simulink model "INtegrated_Simplified_Batteries_2"  (R2025a)
settings: Solver=ode113  StartTime=0.0  StopTime=20000  FixedStep=0.01  MaxStep=0.1  RelTol=1e-3
libraries: simulink x16, slpidlib x2, spsFirstOrderFilterLib x1
(part 1 of 3)
settings Model: Creator=kbiswas  LastModifiedBy=kaust
settings SolverCC: ZeroCrossAlgorithm=Adaptive
settings DebuggingCC: UnderspecifiedInitializationDetection=Classic  MergeDetectMultiDrivingBlocksExec=none
settings ModelReferenceCC: PropagateSignalLabelsOutOfModel=off
settings RTWCC: GPUComputeCapability=3.5

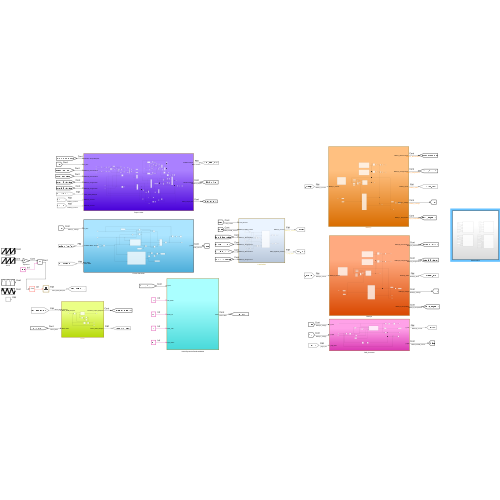
[thumbnail: Simulink's stored preview of the top-level diagram]
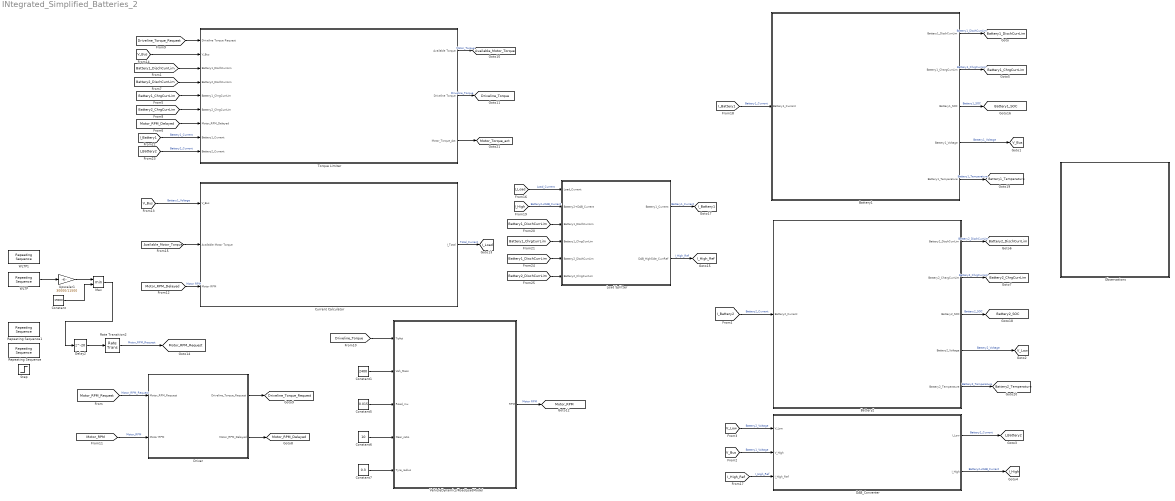
== system INtegrated_Simplified_Batteries_2 ==
  Battery1 : Subsystem
  Battery2 : Subsystem
  Constant : Constant  Value=19000
  Constant1 : Constant  Value=2400
  Constant5 : Constant  Value=0.015
  Constant6 : Constant  Value=10
  Constant7 : Constant  Value=0.3
  Current Calculator : Subsystem
  DAB_Converter : Subsystem
  Delay2 : Delay  DelayLength=20
  Driver : Subsystem
  Load Splitter : Subsystem
  Max : MinMax  Inputs=2
  Observations : Subsystem
  Rate Transition2 : RateTransition
  Repeating Sequence : simulink/Sources/Repeating Sequence  rep_seq_t=[0 20 40 60 80]  rep_seq_y=[0 16000 0 -16000 0]
  Repeating Sequence1 : simulink/Sources/Repeating Sequence  rep_seq_t=[0 0.5 1 2 4 8 16 22 30 38 44 52 56 58 59 59.5 60 64]  rep_seq_y=[0 200 1000 4000 10000 12000 15500 17000 17500 17000 15500 12000 10000 4000 1000 500 0 0]
  Step : Step  Time=2  After=6000  SampleTime=0
  Torque Limiter : Subsystem
  Upscaler1 : Gain  Gain=30000/11500
  VehicleDynamics/RoadLoadModel : Subsystem
  WLTP : simulink/Sources/Repeating Sequence  rep_seq_t=time  rep_seq_y=WLTP_data
  WLTP1 : simulink/Sources/Repeating Sequence  rep_seq_t=time  rep_seq_y=WLTP_data
  tag scope: Available_Motor_Torque=global, Battery1_ChrgCurrLim=global, Battery1_DischCurrLim=global, Battery1_SOC=global, Battery1_Temperature=global, Battery2_ChrgCurrLim=global, Battery2_DischCurrLim=global, Battery2_SOC=global, Battery2_Temperature=global, Driveline_Torque=global, Driveline_Torque_Request=global, I_Battery1=global, I_Battery2=global, I_High=global, I_High_Ref=global, I_Load=global, Motor_RPM=global, Motor_RPM_Delayed=global, Motor_RPM_Request=global, Motor_Torque_act=global, V_Bus=global, V_Low=global
  wires:
  Battery1/1(Battery1_DischCurrLim) -> [Battery1_DischCurrLim]  "Battery1_DischCurrLim"
  Battery1/2(Battery1_ChargCurrLim) -> [Battery1_ChrgCurrLim]  "Battery1_ChrgCurrLim"
  Battery1/4(Battery1_Voltage) -> [V_Bus]  "Battery1_Voltage"
  Battery2/1(Battery2_DischCurrLim) -> [Battery2_DischCurrLim]  "Battery2_DischCurrLim"
  Battery2/2(Battery2_ChargCurrLim) -> [Battery2_ChrgCurrLim]  "Battery2_ChrgCurrLim"
  Battery2/4(Battery2_Voltage) -> [V_Low]  "Battery2_Voltage"
  [I_Battery2] -> Battery2/1(Battery2_Current)  "Battery2_Current"
  [V_Bus] -> DAB_Converter/2(V_High)  "Battery1_Voltage"
  DAB_Converter/1(I_Low) -> [I_Battery2]  "Battery2_Current"
  [V_Low] -> DAB_Converter/1(V_Low)  "Battery2_Voltage"
  [I_Load] -> Load Splitter/1(Load_Current)  "Load_Current"
  DAB_Converter/2(I_High) -> [I_High]  "Battery2+DAB_Current"
  [Motor_RPM_Delayed] -> Current Calculator/3(Motor RPM)  "Motor RPM"
  Torque Limiter/2(Driveline Torque) -> [Driveline_Torque]  "Driveline_Torque"
  [Motor_RPM] -> Driver/2(Motor RPM)  "Motor_RPM"
  [Motor_RPM_Request] -> Driver/1(Motor_RPM_Request)  "Motor_RPM_Request"
  Driver/1(Driveline_Torque_Request) -> [Driveline_Torque_Request]
  [Available_Motor_Torque] -> Current Calculator/2(Available Motor Torque)
  [Battery2_ChrgCurrLim] -> Torque Limiter/6(Battery2_ChrgCurrLim)
  [Driveline_Torque] -> VehicleDynamics/RoadLoadModel/1(TqAct)
  [V_Bus] -> Torque Limiter/2(V_Bus)
  [Battery1_ChrgCurrLim] -> Torque Limiter/5(Battery1_ChrgCurrLim)
  [Battery1_DischCurrLim] -> Torque Limiter/3(Battery1_DischCurrLim)
  [V_Bus] -> Current Calculator/1(V_Bus)  "Battery1_Voltage"
  Constant6/1 -> VehicleDynamics/RoadLoadModel/4(Gear_ratio)
  Constant1/1 -> VehicleDynamics/RoadLoadModel/2(Veh_Mass)
  Constant5/1 -> VehicleDynamics/RoadLoadModel/3(Road_mu)
  [Battery2_DischCurrLim] -> Torque Limiter/4(Battery2_DischCurrLim)
  [Motor_RPM_Delayed] -> Torque Limiter/7(Motor_RPM_Delayed)
  Torque Limiter/1(Available Torque) -> [Available_Motor_Torque]  "Motor_Torque"
  Constant7/1 -> VehicleDynamics/RoadLoadModel/5(Tyre_radius)
  VehicleDynamics/RoadLoadModel/1(RPM) -> [Motor_RPM]  "Motor RPM"
  Driver/2(Motor_RPM_Delayed) -> [Motor_RPM_Delayed]
  Current Calculator/1(I_Total) -> [I_Load]  "Total_Current"
  [Driveline_Torque_Request] -> Torque Limiter/1(Driveline Torque Request)
  Rate Transition2/1 -> [Motor_RPM_Request]  "Motor_RPM_Request"
  Delay2/1 -> Rate Transition2/1
  [I_High_Ref] -> DAB_Converter/3(I_High_Ref)  "I_High_Ref"
  [I_Battery1] -> Battery1/1(Battery1_Current)  "Battery1_Current"
  Load Splitter/1(Battery1_Current) -> [I_Battery1]  "Battery1_Current"
  Load Splitter/2(DAB_HighSide_CurrRef) -> [I_High_Ref]  "I_High_Ref"
  [I_High] -> Load Splitter/2(Battery2+DAB_Current)  "Battery2+DAB_Current"
  [Battery1_DischCurrLim] -> Load Splitter/3(Battery1_DischCurrLim)
  [Battery1_ChrgCurrLim] -> Load Splitter/4(Battery1_ChrgCurrLim)
  Battery1/3(Battery1_SOC) -> [Battery1_SOC]  "Battery1_SOC"
  Battery2/3(Battery2_SOC) -> [Battery2_SOC]  "Battery2_SOC"
  Battery1/5(Battery1_Temperature) -> [Battery1_Temperature]  "Battery1_Temperature"
  Battery2/5(Battery2_Temperature) -> [Battery2_Temperature]  "Battery2_Temperature"
  [I_Battery1] -> Torque Limiter/8(Battery1_Current)  "Battery1_Current"
  [I_Battery2] -> Torque Limiter/9(Battery2_Current)  "Battery2_Current"
  Torque Limiter/3(Motor_Torque_Act) -> [Motor_Torque_act]
  WLTP/1 -> Upscaler1/1
  Constant/1 -> Max/2
  Max/1 -> Delay2/1
  [Battery2_DischCurrLim] -> Load Splitter/6(Battery2_ChrgCurrLim)
  [Battery1_DischCurrLim] -> Load Splitter/5(Battery2_DischCurrLim)
  Upscaler1/1 -> Max/1

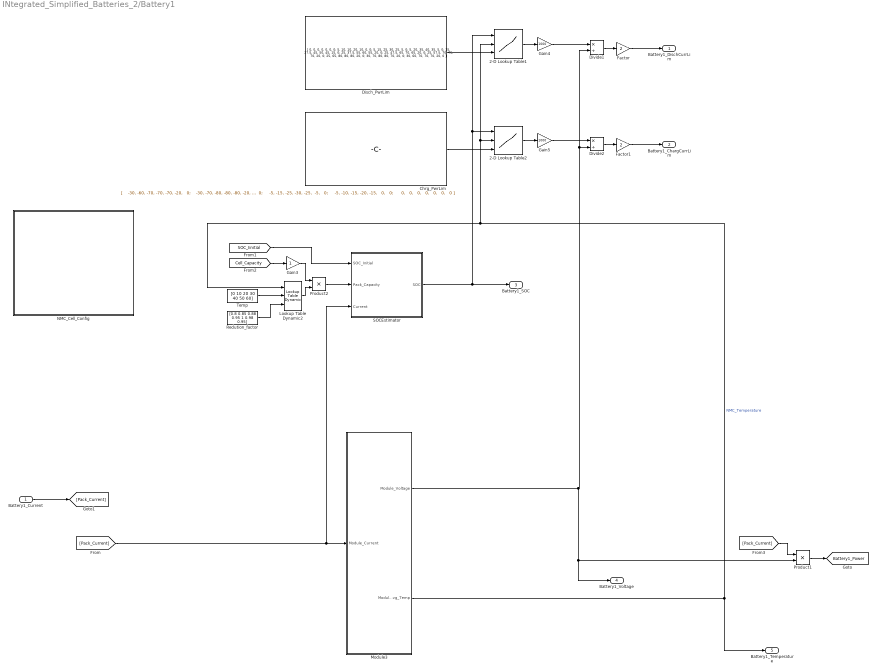
== system INtegrated_Simplified_Batteries_2/Battery1 ==
  Battery1_Current : Inport
  2-D Lookup Table1 : Lookup_n-D  LookupTableObject=''  BreakpointsForDimension1=[0 0.1 0.2 0.3 0.4 0.5 0.6 0.7 0.8 0.9 1]  BreakpointsForDimension2=[0 10 20 30 40 50 60]  BreakpointsForDimension1FirstPoint=10  BreakpointsForDimension2FirstPoint=10  BreakpointsForDimension1Spacing=12  BreakpointsForDimension2Spacing=12  IndexSearchMethod=Evenly spaced points  TableSource=Input port  Table=|  InterpMethod=Akima spline  DiagnosticForOutOfRangeInput=Error  InternalRulePriority=Speed  RndMeth=Simplest
      | [
      |     2.954364, 3.109857, 3.273534, 3.3066, 3.34,    3.3734,  3.20473;
      |     3.122427, 3.286765, 3.459753, 3.4947, 3.53,    3.5653,  3.387035;
      |     3.175499, 3.342631, 3.518559, 3.5541, 3.59,    3.6259,  3.444605;
      |     3.210881, 3.379875, 3.557763, 3.5937, 3.63,    3.6663,  3.482985;
      |     3.237417, 3.407808, 3.587166, 3.6234, 3.66,    3.6966,  3.511777;
      |     3.272799, 3.445052, 3.62637,  3.663,  3.7,     3.737,   3.55015;
      |     3.317026, 3.491066, 3.675375, 3.7125, 3.75,    3.7875,  3.598125;
      |     3.387789, 3.566094, 3.753783, 3.7917, 3.83,    3.8683,  3.674885;
      |     3.467398, 3.649892, 3.841992, 3.8808, 3.92,    3.9592,  3.76124;
      |     3.564697, 3.752313, 3.949803, 3.9897, 4.03,    4.0703,  3.866785;
      |     3.653151, 3.845422, 4.047813, 4.0887, 4.13,    4.1713,  3.962735
      | ]
      settings: InputPortMap=u0,u1,p221
  2-D Lookup Table2 : Lookup_n-D  LookupTableObject=''  BreakpointsForDimension1=[0 0.1 0.2 0.3 0.4 0.5 0.6 0.7 0.8 0.9 1]  BreakpointsForDimension2=[0 10 20 30 40 50 60]  BreakpointsForDimension1FirstPoint=10  BreakpointsForDimension2FirstPoint=10  BreakpointsForDimension1Spacing=12  BreakpointsForDimension2Spacing=12  IndexSearchMethod=Evenly spaced points  TableSource=Input port  Table=|  InterpMethod=Akima spline  DiagnosticForOutOfRangeInput=Error  InternalRulePriority=Speed  RndMeth=Simplest
      | [
      |     2.954364, 3.109857, 3.273534, 3.3066, 3.34,    3.3734,  3.20473;
      |     3.122427, 3.286765, 3.459753, 3.4947, 3.53,    3.5653,  3.387035;
      |     3.175499, 3.342631, 3.518559, 3.5541, 3.59,    3.6259,  3.444605;
      |     3.210881, 3.379875, 3.557763, 3.5937, 3.63,    3.6663,  3.482985;
      |     3.237417, 3.407808, 3.587166, 3.6234, 3.66,    3.6966,  3.511777;
      |     3.272799, 3.445052, 3.62637,  3.663,  3.7,     3.737,   3.55015;
      |     3.317026, 3.491066, 3.675375, 3.7125, 3.75,    3.7875,  3.598125;
      |     3.387789, 3.566094, 3.753783, 3.7917, 3.83,    3.8683,  3.674885;
      |     3.467398, 3.649892, 3.841992, 3.8808, 3.92,    3.9592,  3.76124;
      |     3.564697, 3.752313, 3.949803, 3.9897, 4.03,    4.0703,  3.866785;
      |     3.653151, 3.845422, 4.047813, 4.0887, 4.13,    4.1713,  3.962735
      | ]
      settings: InputPortMap=u0,u1,p221
  Chrg_PwrLim : Constant  Value=|
      | [
      |    -30, -60, -70, -70, -70, -20,   0;
      |    -30, -70, -80, -80, -80, -20,   0;
      |    -25, -65, -80, -80, -80, -20,   0;
      |    -25, -55, -70, -75, -70, -20,   0;
      |    -25, -47.5, -65, -70, -65, -20,  0;
      |    -25, -37.5, -55, -60, -55, -20,  0;
      |    -15, -27.5, -45, -50, -45, -15,  0;
      |     -5, -20, -35, -40, -35,  -5,   0;
      |     -5, -15, -25, -30, -25,  -5,   0;
      |     -5, -10, -15, -20, -15,   0,   0;
      |      0,   0,   0,   0,   0,   0,   0
      | ]
  Disch_PwrLim : Constant  Value=|
      | [
      |      0,   0,   0,   0,   0,   0,   0;
      |      5,  10,  10,  20,  10,   0,   0;
      |      5,  15,  25,  30,  25,   5,   0;
      |      5,  20,  35,  40,  35,   5,   0;
      |     15, 27.5, 45,  50,  45,  15,   0;
      |     25, 37.5, 55,  60,  55,  20,   0;
      |     25, 47.5, 65,  70,  65,  20,   0;
      |     25, 57.5, 70,  75,  70,  20,   0;
      |     25, 65,   80,  80,  80,  20,   0;
      |     30, 70,   80,  80,  70,  20,   0;
      |     30, 60,   70,  70,  70,  20,   0
      | ]
  Divide1 : Product  Inputs=*/
  Divide2 : Product  Inputs=*/
  Factor : Gain  Gain=2
  Factor1 : Gain  Gain=2
  Gain3 : Gain
  Gain4 : Gain  Gain=1000
  Gain5 : Gain  Gain=1000
  Lookup Table Dynamic2 : simulink/Lookup Tables/Lookup Table Dynamic  LookUpMeth=Interpolation-Use End Values  OutDataType=fixdt('double')  OutScaling=[]  OutputDataTypeScalingMode=Specify via dialog  OutDataTypeStr=fixdt('double')  DoSatur=off
  Module3 : Subsystem
  NMC_Cell_Config : Subsystem
  Product1 : Product
  Product2 : Product
  Redution_factor : Constant  Value=[0.8 0.85 0.88 0.95 1 0.98 0.95]
  SOCEstimator : Subsystem  TreatAsAtomicUnit=on
  Temp : Constant  Value=[0 10 20 30 40 50 60]
  Battery1_DischCurrLim : Outport
  Battery1_ChargCurrLim : Outport  Port=2
  Battery1_SOC : Outport  Port=3
  Battery1_Voltage : Outport  Port=4
  Battery1_Temperature : Outport  Port=5
  tag scope: Battery1_Power=global
  wires:
  Product2/1 -> SOCEstimator/2(Pack_Capacity)
  [Pack_Current] -> SOCEstimator/3(Current), Module3/1(Module_Current)
  Divide1/1 -> Factor/1
  Module3/2(Module_avg_Temp) -> Battery1_Temperature/1, 2-D Lookup Table1/2, 2-D Lookup Table2/2, Lookup Table Dynamic2/1  "NMC_Temperature"
  Lookup Table Dynamic2/1 -> Product2/2
  Temp/1 -> Lookup Table Dynamic2/2
  Module3/1(Module_Voltage) -> Divide1/2, Divide2/2, Battery1_Voltage/1, Product1/2
  SOCEstimator/1(SOC) -> Battery1_SOC/1, 2-D Lookup Table2/1, 2-D Lookup Table1/1
  Gain4/1 -> Divide1/1
  2-D Lookup Table1/1 -> Gain4/1
  [SOC_Iinitial] -> SOCEstimator/1(SOC_Initial)
  Divide2/1 -> Factor1/1
  Disch_PwrLim/1 -> 2-D Lookup Table1/3
  2-D Lookup Table2/1 -> Gain5/1
  [Cell_Capacity] -> Gain3/1
  Redution_factor/1 -> Lookup Table Dynamic2/3
  Chrg_PwrLim/1 -> 2-D Lookup Table2/3
  Gain3/1 -> Product2/1
  Gain5/1 -> Divide2/1
  Battery1_Current/1 -> [Pack_Current]
  Factor/1 -> Battery1_DischCurrLim/1
  Factor1/1 -> Battery1_ChargCurrLim/1
  [Pack_Current] -> Product1/1
  Product1/1 -> [Battery1_Power]

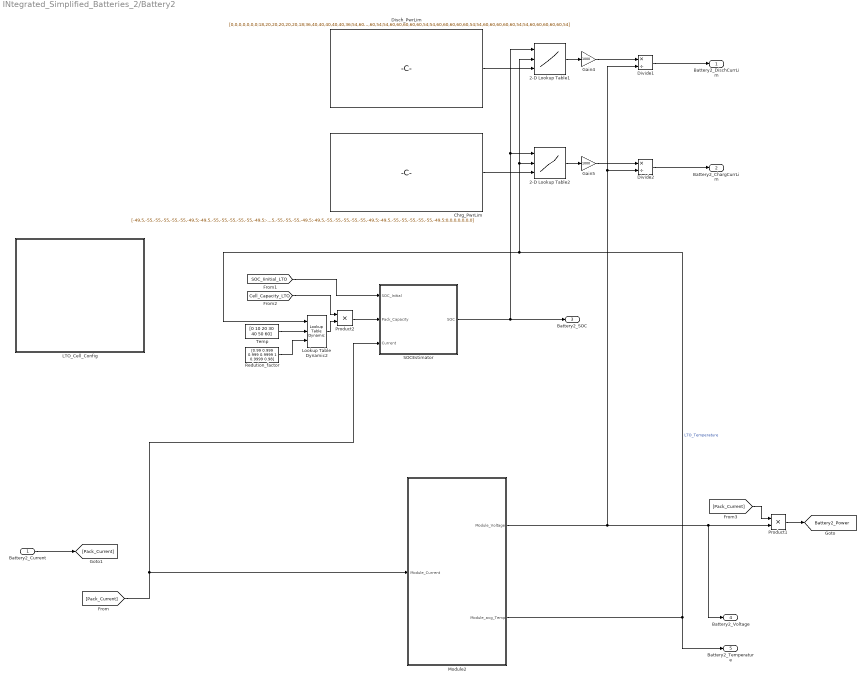
== system INtegrated_Simplified_Batteries_2/Battery2 ==
  Battery2_Current : Inport
  2-D Lookup Table1 : Lookup_n-D  LookupTableObject=''  BreakpointsForDimension1=[0 0.1 0.2 0.3 0.4 0.5 0.6 0.7 0.8 0.9 1]  BreakpointsForDimension2=[0 10 20 30 40 50 60]  BreakpointsForDimension1FirstPoint=10  BreakpointsForDimension2FirstPoint=10  BreakpointsForDimension1Spacing=12  BreakpointsForDimension2Spacing=12  IndexSearchMethod=Evenly spaced points  TableSource=Input port  Table=|  InterpMethod=Akima spline  InternalRulePriority=Speed  RndMeth=Simplest
      | [
      |     2.954364, 3.109857, 3.273534, 3.3066, 3.34,    3.3734,  3.20473;
      |     3.122427, 3.286765, 3.459753, 3.4947, 3.53,    3.5653,  3.387035;
      |     3.175499, 3.342631, 3.518559, 3.5541, 3.59,    3.6259,  3.444605;
      |     3.210881, 3.379875, 3.557763, 3.5937, 3.63,    3.6663,  3.482985;
      |     3.237417, 3.407808, 3.587166, 3.6234, 3.66,    3.6966,  3.511777;
      |     3.272799, 3.445052, 3.62637,  3.663,  3.7,     3.737,   3.55015;
      |     3.317026, 3.491066, 3.675375, 3.7125, 3.75,    3.7875,  3.598125;
      |     3.387789, 3.566094, 3.753783, 3.7917, 3.83,    3.8683,  3.674885;
      |     3.467398, 3.649892, 3.841992, 3.8808, 3.92,    3.9592,  3.76124;
      |     3.564697, 3.752313, 3.949803, 3.9897, 4.03,    4.0703,  3.866785;
      |     3.653151, 3.845422, 4.047813, 4.0887, 4.13,    4.1713,  3.962735
      | ]
      settings: InputPortMap=u0,u1,p221
  2-D Lookup Table2 : Lookup_n-D  LookupTableObject=''  BreakpointsForDimension1=[0 0.1 0.2 0.3 0.4 0.5 0.6 0.7 0.8 0.9 1]  BreakpointsForDimension2=[0 10 20 30 40 50 60]  BreakpointsForDimension1FirstPoint=10  BreakpointsForDimension2FirstPoint=10  BreakpointsForDimension1Spacing=12  BreakpointsForDimension2Spacing=12  IndexSearchMethod=Evenly spaced points  TableSource=Input port  Table=|  InterpMethod=Akima spline  InternalRulePriority=Speed  RndMeth=Simplest
      | [
      |     2.954364, 3.109857, 3.273534, 3.3066, 3.34,    3.3734,  3.20473;
      |     3.122427, 3.286765, 3.459753, 3.4947, 3.53,    3.5653,  3.387035;
      |     3.175499, 3.342631, 3.518559, 3.5541, 3.59,    3.6259,  3.444605;
      |     3.210881, 3.379875, 3.557763, 3.5937, 3.63,    3.6663,  3.482985;
      |     3.237417, 3.407808, 3.587166, 3.6234, 3.66,    3.6966,  3.511777;
      |     3.272799, 3.445052, 3.62637,  3.663,  3.7,     3.737,   3.55015;
      |     3.317026, 3.491066, 3.675375, 3.7125, 3.75,    3.7875,  3.598125;
      |     3.387789, 3.566094, 3.753783, 3.7917, 3.83,    3.8683,  3.674885;
      |     3.467398, 3.649892, 3.841992, 3.8808, 3.92,    3.9592,  3.76124;
      |     3.564697, 3.752313, 3.949803, 3.9897, 4.03,    4.0703,  3.866785;
      |     3.653151, 3.845422, 4.047813, 4.0887, 4.13,    4.1713,  3.962735
      | ]
      settings: InputPortMap=u0,u1,p221
  Chrg_PwrLim : Constant  Value=[-49.5,-55,-55,-55,-55,-55,-49.5;-49.5,-55,-55,-55,-55,-55,-49.5;-49.5,-55,-55,-55,-55,-55,-49.5;-49.5,-55,-55,-55,-55,-55,-49.5;-49.5,-55,-55,-55,-55,-55,-49.5;-49.5,-55,-55,-55,-55,-55,-49.5;-49.5,-55,-55,-55,-55,-55,-49.5;-49.5,-55,-55,-55,-55,-55,-49.5;-49.5,-55,-55,-55,-55,-55,-49.5;-49.5,-55,-55,-55,-55,-55,-49.5;0,0,0,0,0,0,0]
  Disch_PwrLim : Constant  Value=[0,0,0,0,0,0,0;18,20,20,20,20,20,18;36,40,40,40,40,40,36;54,60,60,60,60,60,54;54,60,60,60,60,60,54;54,60,60,60,60,60,54;54,60,60,60,60,60,54;54,60,60,60,60,60,54;54,60,60,60,60,60,54;54,60,60,60,60,60,54;54,60,60,60,60,60,54]
  Divide1 : Product  Inputs=*/
  Divide2 : Product  Inputs=*/
  Gain4 : Gain  Gain=1000
  Gain5 : Gain  Gain=1000
  LTO_Cell_Config : Subsystem
  Lookup Table Dynamic2 : simulink/Lookup Tables/Lookup Table Dynamic  LookUpMeth=Interpolation-Use End Values  OutDataType=fixdt('double')  OutScaling=[]  OutputDataTypeScalingMode=Specify via dialog  OutDataTypeStr=fixdt('double')  DoSatur=off
  Module2 : Subsystem
  Product1 : Product
  Product2 : Product
  Redution_factor : Constant  Value=[0.99 0.999 0.999 0.9999 1 0.9999 0.98]
  SOCEstimator : Subsystem  TreatAsAtomicUnit=on
  Temp : Constant  Value=[0 10 20 30 40 50 60]
  Battery2_DischCurrLim : Outport
  Battery2_ChargCurrLim : Outport  Port=2
  Battery2_SOC : Outport  Port=3
  Battery2_Voltage : Outport  Port=4
  Battery2_Temperature : Outport  Port=5
  tag scope: Battery2_Power=global
  wires:
  Product2/1 -> SOCEstimator/2(Pack_Capacity)
  Divide1/1 -> Battery2_DischCurrLim/1
  Module2/2(Module_avg_Temp) -> Battery2_Temperature/1, 2-D Lookup Table1/2, 2-D Lookup Table2/2, Lookup Table Dynamic2/1  "LTO_Temperature"
  Lookup Table Dynamic2/1 -> Product2/2
  Temp/1 -> Lookup Table Dynamic2/2
  SOCEstimator/1(SOC) -> Battery2_SOC/1, 2-D Lookup Table2/1, 2-D Lookup Table1/1
  Gain4/1 -> Divide1/1
  2-D Lookup Table1/1 -> Gain4/1
  [SOC_Iinitial_LTO] -> SOCEstimator/1(SOC_Initial)
  Divide2/1 -> Battery2_ChargCurrLim/1
  Disch_PwrLim/1 -> 2-D Lookup Table1/3
  2-D Lookup Table2/1 -> Gain5/1
  Redution_factor/1 -> Lookup Table Dynamic2/3
  Chrg_PwrLim/1 -> 2-D Lookup Table2/3
  [Cell_Capacity_LTO] -> Product2/1
  Gain5/1 -> Divide2/1
  Battery2_Current/1 -> [Pack_Current]
  [Pack_Current] -> Module2/1(Module_Current), SOCEstimator/3(Current)
  Module2/1(Module_Voltage) -> Battery2_Voltage/1, Product1/2, Divide2/2, Divide1/2
  [Pack_Current] -> Product1/1
  Product1/1 -> [Battery2_Power]

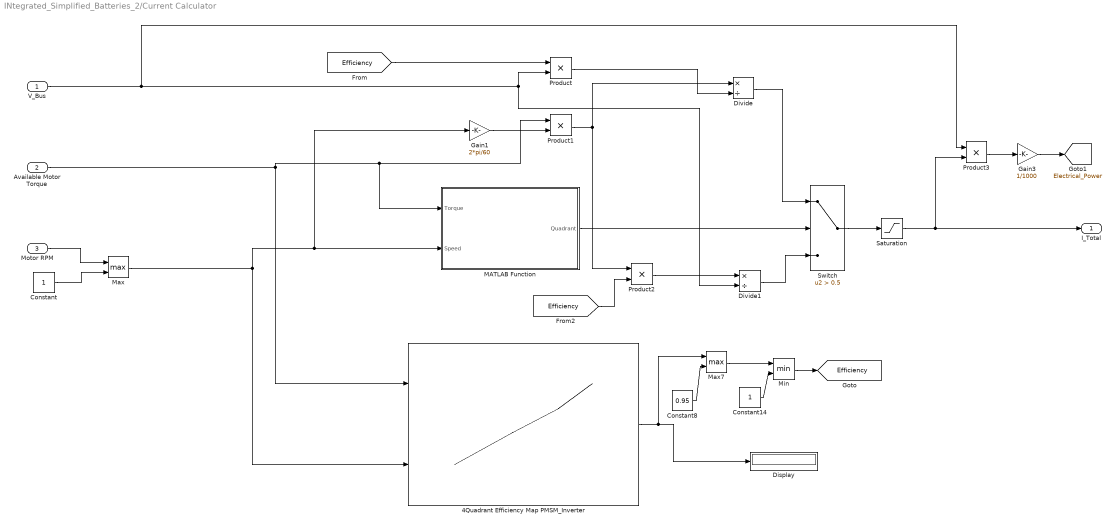
== system INtegrated_Simplified_Batteries_2/Current Calculator ==
  V_Bus : Inport
  Available Motor Torque : Inport  Port=2
  Motor RPM : Inport  Port=3
  4Quadrant Efficiency Map PMSM_Inverter : Lookup_n-D  BreakpointsForDimension1=-200:20:200  BreakpointsForDimension2=-16000:500:16000  Table=|  InterpMethod=Akima spline  InternalRulePriority=Speed  RndMeth=Simplest
      | [0.9785 0.9788 0.9792 0.9795 0.9799 0.9800 0.9800 0.9800 0.9800 0.9800 0.9800 0.9800 0.9800 0.9800 0.9800 0.9800 0.9800 0.9800 0.9800 0.9800 0.9800 0.9800 0.9800 0.9794 0.9781 0.9762 0.9737 0.9699 0.9641 0.9542 0.9347 0.8797 0.0000 0.8632 0.9301 0.9520 0.9628 0.9690 0.9730 0.9757 0.9776 0.9789 0.9799 0.9800 0.9800 0.9800 0.9800 0.9800 0.9800 0.9800 0.9800 0.9800 0.9800 0.9800 0.9800 0.9800 0.9800 0.9800 0.9800 0.9798 0.9794 0.9791 0.9787 0.9784 0.9780;
      | 0.9770 0.9774 0.9778 0.9782 0.9786 0.9790 0.9794 0.9797 0.9800 0.9800 0.9800 0.9800 0.9800 0.9800 0.9800 0.9800 0.9800 0.9800 0.9800 0.9800 0.9800 0.9800 0.9800 0.9800 0.9790 0.9774 0.9752 0.9719 0.9667 0.9578 0.9400 0.8894 0.0000 0.8756 0.9361 0.9559 0.9655 0.9711 0.9746 0.9769 0.9785 0.9797 0.9800 0.9800 0.9800 0.9800 0.9800 0.9800 0.9800 0.9800 0.9800 0.9800 0.9800 0.9800 0.9800 0.9797 0.9793 0.9789 0.9785 0.9781 0.9777 0.9773 0.9769 0.9764 0.9764;
      | 0.9750 0.9755 0.9760 0.9765 0.9769 0.9774 0.9779 0.9783 0.9787 0.9792 0.9796 0.9799 0.9800 0.9800 0.9800 0.9800 0.9800 0.9800 0.9800 0.9800 0.9800 0.9800 0.9800 0.9800 0.9797 0.9785 0.9766 0.9737 0.9691 0.9612 0.9452 0.8992 0.0000 0.8878 0.9420 0.9596 0.9681 0.9730 0.9760 0.9780 0.9793 0.9800 0.9800 0.9800 0.9800 0.9800 0.9800 0.9800 0.9800 0.9800 0.9800 0.9800 0.9799 0.9795 0.9791 0.9787 0.9783 0.9778 0.9774 0.9769 0.9764 0.9759 0.9754 0.9749 0.9743;
      | 0.9723 0.9729 0.9735 0.9741 0.9747 0.9752 0.9758 0.9764 0.9769 0.9774 0.9779 0.9784 0.9789 0.9793 0.9798 0.9800 0.9800 0.9800 0.9800 0.9800 0.9800 0.9800 0.9800 0.9800 0.9800 0.9793 0.9778 0.9754 0.9714 0.9645 0.9503 0.9089 0.0000 0.8998 0.9477 0.9632 0.9706 0.9747 0.9772 0.9788 0.9799 0.9800 0.9800 0.9800 0.9800 0.9800 0.9800 0.9800 0.9800 0.9798 0.9794 0.9789 0.9784 0.9779 0.9774 0.9769 0.9763 0.9758 0.9752 0.9746 0.9740 0.9734 0.9728 0.9722 0.9716;
      | 0.9687 0.9694 0.9701 0.9708 0.9715 0.9722 0.9729 0.9736 0.9743 0.9749 0.9756 0.9762 0.9768 0.9774 0.9780 0.9785 0.9790 0.9795 0.9799 0.9800 0.9800 0.9800 0.9800 0.9800 0.9800 0.9798 0.9786 0.9767 0.9735 0.9676 0.9553 0.9186 0.0000 0.9114 0.9532 0.9665 0.9728 0.9762 0.9782 0.9794 0.9800 0.9800 0.9800 0.9800 0.9800 0.9799 0.9795 0.9791 0.9786 0.9780 0.9775 0.9769 0.9763 0.9756 0.9750 0.9743 0.9736 0.9729 0.9722 0.9714 0.9707 0.9700 0.9692 0.9685 0.9677;
      | 0.9635 0.9644 0.9653 0.9661 0.9670 0.9679 0.9687 0.9696 0.9704 0.9712 0.9721 0.9729 0.9737 0.9744 0.9752 0.9759 0.9767 0.9773 0.9780 0.9786 0.9791 0.9795 0.9798 0.9800 0.9800 0.9798 0.9790 0.9777 0.9751 0.9703 0.9598 0.9280 0.0000 0.9224 0.9582 0.9694 0.9745 0.9772 0.9786 0.9793 0.9796 0.9796 0.9794 0.9791 0.9786 0.9781 0.9775 0.9768 0.9761 0.9753 0.9746 0.9738 0.9730 0.9721 0.9713 0.9704 0.9695 0.9686 0.9677 0.9668 0.9659 0.9649 0.9640 0.9631 0.9621;
      | 0.9557 0.9568 0.9579 0.9590 0.9601 0.9611 0.9622 0.9633 0.9644 0.9655 0.9666 0.9676 0.9687 0.9697 0.9707 0.9717 0.9727 0.9737 0.9746 0.9755 0.9763 0.9771 0.9777 0.9783 0.9787 0.9788 0.9786 0.9778 0.9761 0.9723 0.9638 0.9367 0.0000 0.9324 0.9624 0.9715 0.9755 0.9773 0.9781 0.9784 0.9782 0.9778 0.9772 0.9765 0.9757 0.9749 0.9739 0.9730 0.9720 0.9709 0.9699 0.9688 0.9677 0.9665 0.9654 0.9643 0.9631 0.9619 0.9608 0.9596 0.9584 0.9572 0.9560 0.9548 0.9536;
      | 0.9426 0.9440 0.9455 0.9470 0.9484 0.9499 0.9513 0.9528 0.9543 0.9557 0.9572 0.9586 0.9601 0.9615 0.9629 0.9643 0.9657 0.9671 0.9685 0.9698 0.9710 0.9723 0.9734 0.9745 0.9754 0.9761 0.9765 0.9764 0.9755 0.9730 0.9663 0.9438 0.0000 0.9404 0.9651 0.9722 0.9749 0.9759 0.9759 0.9755 0.9748 0.9738 0.9727 0.9715 0.9702 0.9688 0.9674 0.9660 0.9645 0.9630 0.9615 0.9600 0.9584 0.9568 0.9553 0.9537 0.9521 0.9505 0.9489 0.9472 0.9456 0.9440 0.9424 0.9407 0.9391;
      | 0.9171 0.9192 0.9213 0.9234 0.9256 0.9277 0.9298 0.9320 0.9341 0.9363 0.9384 0.9406 0.9427 0.9449 0.9470 0.9492 0.9513 0.9534 0.9555 0.9576 0.9597 0.9617 0.9637 0.9656 0.9673 0.9689 0.9703 0.9712 0.9714 0.9701 0.9653 0.9463 0.0000 0.9433 0.9640 0.9692 0.9706 0.9703 0.9694 0.9679 0.9662 0.9643 0.9623 0.9602 0.9580 0.9558 0.9535 0.9512 0.9488 0.9464 0.9441 0.9417 0.9392 0.9368 0.9344 0.9319 0.9295 0.9270 0.9245 0.9221 0.9196 0.9171 0.9146 0.9121 0.9096;
      | 0.8478 0.8514 0.8551 0.8588 0.8625 0.8662 0.8700 0.8738 0.8776 0.8815 0.8854 0.8893 0.8932 0.8972 0.9011 0.9051 0.9091 0.9132 0.9172 0.9213 0.9253 0.9293 0.9333 0.9372 0.9410 0.9447 0.9481 0.9510 0.9532 0.9537 0.9502 0.9309 0.0000 0.9257 0.9476 0.9515 0.9509 0.9485 0.9452 0.9415 0.9373 0.9330 0.9285 0.9239 0.9193 0.9145 0.9097 0.9049 0.9001 0.8952 0.8903 0.8854 0.8804 0.8755 0.8705 0.8655 0.8606 0.8556 0.8506 0.8456 0.8406 0.8356 0.8305 0.8255 0.8205;
      | 0.0000 0.0000 0.0000 0.0000 0.0000 0.0000 0.0000 0.0000 0.0000 0.0000 0.0000 0.0000 0.0000 0.0000 0.0000 0.0000 0.0000 0.0000 0.0000 0.0000 0.0000 0.0000 0.0000 0.0000 0.0000 0.0000 0.0000 0.0000 0.0000 0.0000 0.0000 0.0000 0.0000 0.0000 0.0000 0.0000 0.0000 0.0000 0.0000 0.0000 0.0000 0.0000 0.0000 0.0000 0.0000 0.0000 0.0000 0.0000 0.0000 0.0000 0.0000 0.0000 0.0000 0.0000 0.0000 0.0000 0.0000 0.0000 0.0000 0.0000 0.0000 0.0000 0.0000 0.0000 0.0000;
      | 0.8205 0.8255 0.8305 0.8356 0.8406 0.8456 0.8506 0.8556 0.8606 0.8655 0.8705 0.8755 0.8804 0.8854 0.8903 0.8952 0.9001 0.9049 0.9097 0.9145 0.9193 0.9239 0.9285 0.9330 0.9373 0.9415 0.9452 0.9485 0.9509 0.9515 0.9476 0.9257 0.0000 0.9309 0.9502 0.9537 0.9532 0.9510 0.9481 0.9447 0.9410 0.9372 0.9333 0.9293 0.9253 0.9213 0.9172 0.9132 0.9091 0.9051 0.9011 0.8972 0.8932 0.8893 0.8854 0.8815 0.8776 0.8738 0.8700 0.8662 0.8625 0.8588 0.8551 0.8514 0.8478;
      | 0.9096 0.9121 0.9146 0.9171 0.9196 0.9221 0.9245 0.9270 0.9295 0.9319 0.9344 0.9368 0.9392 0.9417 0.9441 0.9464 0.9488 0.9512 0.9535 0.9558 0.9580 0.9602 0.9623 0.9643 0.9662 0.9679 0.9694 0.9703 0.9706 0.9692 0.9640 0.9433 0.0000 0.9463 0.9653 0.9701 0.9714 0.9712 0.9703 0.9689 0.9673 0.9656 0.9637 0.9617 0.9597 0.9576 0.9555 0.9534 0.9513 0.9492 0.9470 0.9449 0.9427 0.9406 0.9384 0.9363 0.9341 0.9320 0.9298 0.9277 0.9256 0.9234 0.9213 0.9192 0.9171;
      | 0.9391 0.9407 0.9424 0.9440 0.9456 0.9472 0.9489 0.9505 0.9521 0.9537 0.9553 0.9568 0.9584 0.9600 0.9615 0.9630 0.9645 0.9660 0.9674 0.9688 0.9702 0.9715 0.9727 0.9738 0.9748 0.9755 0.9759 0.9759 0.9749 0.9722 0.9651 0.9404 0.0000 0.9438 0.9663 0.9730 0.9755 0.9764 0.9765 0.9761 0.9754 0.9745 0.9734 0.9723 0.9710 0.9698 0.9685 0.9671 0.9657 0.9643 0.9629 0.9615 0.9601 0.9586 0.9572 0.9557 0.9543 0.9528 0.9513 0.9499 0.9484 0.9470 0.9455 0.9440 0.9426;
      | 0.9536 0.9548 0.9560 0.9572 0.9584 0.9596 0.9608 0.9619 0.9631 0.9643 0.9654 0.9665 0.9677 0.9688 0.9699 0.9709 0.9720 0.9730 0.9739 0.9749 0.9757 0.9765 0.9772 0.9778 0.9782 0.9784 0.9781 0.9773 0.9755 0.9715 0.9624 0.9324 0.0000 0.9367 0.9638 0.9723 0.9761 0.9778 0.9786 0.9788 0.9787 0.9783 0.9777 0.9771 0.9763 0.9755 0.9746 0.9737 0.9727 0.9717 0.9707 0.9697 0.9687 0.9676 0.9666 0.9655 0.9644 0.9633 0.9622 0.9611 0.9601 0.9590 0.9579 0.9568 0.9557;
      | 0.9621 0.9631 0.9640 0.9649 0.9659 0.9668 0.9677 0.9686 0.9695 0.9704 0.9713 0.9721 0.9730 0.9738 0.9746 0.9753 0.9761 0.9768 0.9775 0.9781 0.9786 0.9791 0.9794 0.9796 0.9796 0.9793 0.9786 0.9772 0.9745 0.9694 0.9582 0.9224 0.0000 0.9280 0.9598 0.9703 0.9751 0.9777 0.9790 0.9798 0.9800 0.9800 0.9798 0.9795 0.9791 0.9786 0.9780 0.9773 0.9767 0.9759 0.9752 0.9744 0.9737 0.9729 0.9721 0.9712 0.9704 0.9696 0.9687 0.9679 0.9670 0.9661 0.9653 0.9644 0.9635;
      | 0.9677 0.9685 0.9692 0.9700 0.9707 0.9714 0.9722 0.9729 0.9736 0.9743 0.9750 0.9756 0.9763 0.9769 0.9775 0.9780 0.9786 0.9791 0.9795 0.9799 0.9800 0.9800 0.9800 0.9800 0.9800 0.9794 0.9782 0.9762 0.9728 0.9665 0.9532 0.9114 0.0000 0.9186 0.9553 0.9676 0.9735 0.9767 0.9786 0.9798 0.9800 0.9800 0.9800 0.9800 0.9800 0.9800 0.9799 0.9795 0.9790 0.9785 0.9780 0.9774 0.9768 0.9762 0.9756 0.9749 0.9743 0.9736 0.9729 0.9722 0.9715 0.9708 0.9701 0.9694 0.9687;
      | 0.9716 0.9722 0.9728 0.9734 0.9740 0.9746 0.9752 0.9758 0.9763 0.9769 0.9774 0.9779 0.9784 0.9789 0.9794 0.9798 0.9800 0.9800 0.9800 0.9800 0.9800 0.9800 0.9800 0.9800 0.9799 0.9788 0.9772 0.9747 0.9706 0.9632 0.9477 0.8998 0.0000 0.9089 0.9503 0.9645 0.9714 0.9754 0.9778 0.9793 0.9800 0.9800 0.9800 0.9800 0.9800 0.9800 0.9800 0.9800 0.9800 0.9800 0.9798 0.9793 0.9789 0.9784 0.9779 0.9774 0.9769 0.9764 0.9758 0.9752 0.9747 0.9741 0.9735 0.9729 0.9723;
      | 0.9743 0.9749 0.9754 0.9759 0.9764 0.9769 0.9774 0.9778 0.9783 0.9787 0.9791 0.9795 0.9799 0.9800 0.9800 0.9800 0.9800 0.9800 0.9800 0.9800 0.9800 0.9800 0.9800 0.9800 0.9793 0.9780 0.9760 0.9730 0.9681 0.9596 0.9420 0.8878 0.0000 0.8992 0.9452 0.9612 0.9691 0.9737 0.9766 0.9785 0.9797 0.9800 0.9800 0.9800 0.9800 0.9800 0.9800 0.9800 0.9800 0.9800 0.9800 0.9800 0.9800 0.9799 0.9796 0.9792 0.9787 0.9783 0.9779 0.9774 0.9769 0.9765 0.9760 0.9755 0.9750;
      | 0.9764 0.9769 0.9773 0.9777 0.9781 0.9785 0.9789 0.9793 0.9797 0.9800 0.9800 0.9800 0.9800 0.9800 0.9800 0.9800 0.9800 0.9800 0.9800 0.9800 0.9800 0.9800 0.9800 0.9797 0.9785 0.9769 0.9746 0.9711 0.9655 0.9559 0.9361 0.8756 0.0000 0.8894 0.9400 0.9578 0.9667 0.9719 0.9752 0.9774 0.9790 0.9800 0.9800 0.9800 0.9800 0.9800 0.9800 0.9800 0.9800 0.9800 0.9800 0.9800 0.9800 0.9800 0.9800 0.9800 0.9800 0.9797 0.9794 0.9790 0.9786 0.9782 0.9778 0.9774 0.9770;
      | 0.9780 0.9784 0.9787 0.9791 0.9794 0.9798 0.9800 0.9800 0.9800 0.9800 0.9800 0.9800 0.9800 0.9800 0.9800 0.9800 0.9800 0.9800 0.9800 0.9800 0.9800 0.9800 0.9799 0.9789 0.9776 0.9757 0.9730 0.9690 0.9628 0.9520 0.9301 0.8632 0.0000 0.8797 0.9347 0.9542 0.9641 0.9699 0.9737 0.9762 0.9781 0.9794 0.9800 0.9800 0.9800 0.9800 0.9800 0.9800 0.9800 0.9800 0.9800 0.9800 0.9800 0.9800 0.9800 0.9800 0.9800 0.9800 0.9800 0.9800 0.9799 0.9795 0.9792 0.9788 0.9785];
      settings: InputPortMap=u0,u1
  Constant : Constant
  Constant14 : Constant
  Constant8 : Constant  Value=0.95
  Display : Display
  Divide : Product  Inputs=*/
  Divide1 : Product  Inputs=*/
  Gain1 : Gain  Gain=2*pi/60
  Gain3 : Gain  Gain=1/1000
  MATLAB Function : MATLAB Function  TreatAsAtomicUnit=on
  Max : MinMax  Function=max  Inputs=2
  Max7 : MinMax  Function=max  Inputs=2
  Min : MinMax  Inputs=2
  Product{,1..3} (4 alike) : Product
  Saturation : Saturate  UpperLimit=400  LowerLimit=-400
  Switch : Switch  Criteria=u2 > Threshold  Threshold=0.5  SaturateOnIntegerOverflow=off  InputSameDT=off
  I_Total : Outport
  tag scope: Efficiency=global, Electrical_Power=global
  wires:
  [Efficiency] -> Product2/2
  Min/1 -> [Efficiency]
  Max/1 -> Gain1/1, MATLAB Function/2(Speed), 4Quadrant Efficiency Map PMSM_Inverter/2
  4Quadrant Efficiency Map PMSM_Inverter/1 -> Max7/1, Display/1
  Max7/1 -> Min/1
  V_Bus/1 -> Product3/1, Product/2, Divide1/2
  Divide/1 -> Switch/1
  Constant14/1 -> Min/2
  [Efficiency] -> Product/1
  Saturation/1 -> Product3/2, I_Total/1
  Available Motor Torque/1 -> Product1/1, MATLAB Function/1(Torque), 4Quadrant Efficiency Map PMSM_Inverter/1
  Constant8/1 -> Max7/2
  Switch/1 -> Saturation/1
  MATLAB Function/1(Quadrant) -> Switch/2
  Product2/1 -> Divide1/1
  Gain1/1 -> Product1/2
  Product1/1 -> Product2/1, Divide/1
  Divide1/1 -> Switch/3
  Product/1 -> Divide/2
  Product3/1 -> Gain3/1
  Gain3/1 -> [Electrical_Power]
  Motor RPM/1 -> Max/1
  Constant/1 -> Max/2

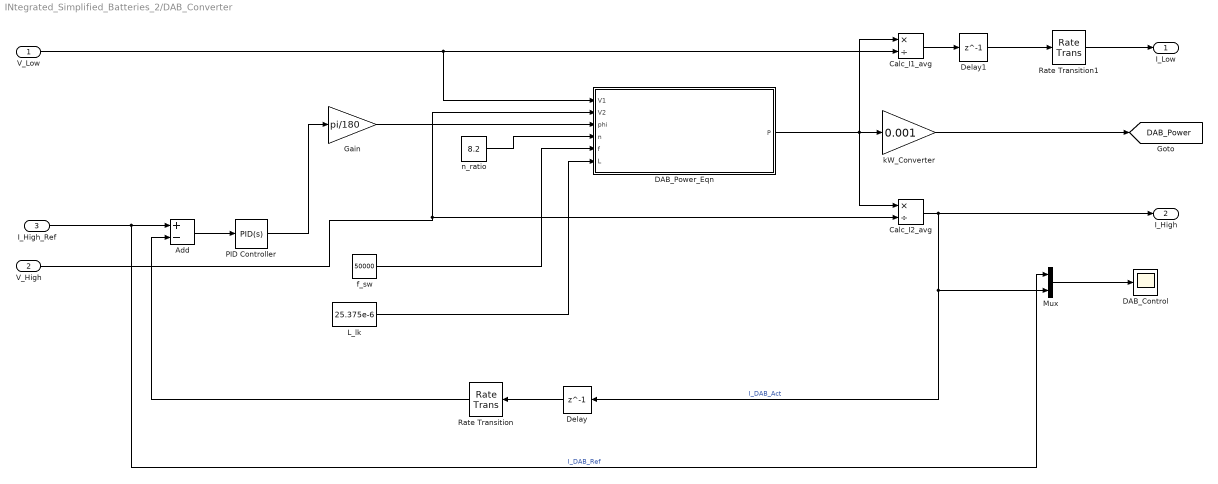
== system INtegrated_Simplified_Batteries_2/DAB_Converter ==
  V_Low : Inport
  V_High : Inport  Port=2
  I_High_Ref : Inport  Port=3
  Add : Sum  Inputs=+-
  Calc_I1_avg : Product  Inputs=*/
  Calc_I2_avg : Product  Inputs=*/
  DAB_Control : Scope
      settings: DataLoggingVariableName=ScopeData8
  DAB_Power_Eqn : MATLAB Function  TreatAsAtomicUnit=on
  Delay : Delay  DelayLength=1
  Delay1 : Delay  DelayLength=1
  Gain : Gain  Gain=pi/180
  L_lk : Constant  Value=25.375e-6
  Mux : Mux  Inputs=2
  PID Controller : slpidlib/PID Controller  Controller=PID  Form=Parallel  TimeDomain=Continuous-time  UseExternalTs=off  SampleTime=-1  IntegratorMethod=Trapezoidal  FilterMethod=Trapezoidal  ControllerParametersSource=internal  P=0.19858489755752  I=0.958995137726395  UseKiTs=off  D=-0.0702303433254038  UseExternalDerivativeSource=off  N=2.71004916651033  UseFilter=on  TunerSelectOption=Transfer Function Based (PID Tuner App)  InitialConditionSource=internal  InitialConditionForIntegrator=0  InitialConditionForFilter=0  DifferentiatorICPrevScaledInput=0  ExternalReset=none  TrackingMode=off  Kt=0.5  LimitOutput=on  SatLimitsSource=internal  UpperSaturationLimit=90  LowerSaturationLimit=-90  LinearizeAsGain=on  AntiWindupMode=back-calculation  Kb=0.5  LimitIntegrator=on  UpperIntegratorSaturationLimit=90  LowerIntegratorSaturationLimit=-90  POutMin=[]  POutMax=[]  IOutMin=[]  IOutMax=[]  DOutMin=[]  DOutMax=[]  NOutMin=[]  NOutMax=[]  SumOutMin=[]  SumOutMax=[]  SaturationOutMin=[]  SaturationOutMax=[]  PParamMin=[]  PParamMax=[]  IParamMin=[]  IParamMax=[]  DParamMin=[]  DParamMax=[]  NParamMin=[]  NParamMax=[]  KbParamMin=[]  KbParamMax=[]  KtParamMin=[]  KtParamMax=[]  KbOutMin=[]  KbOutMax=[]  KtOutMin=[]  KtOutMax=[]  IntegratorOutMin=[]  IntegratorOutMax=[]  FilterOutMin=[]  FilterOutMax=[]  SumI1OutMin=[]  SumI1OutMax=[]  SumI2OutMin=[]  SumI2OutMax=[]  SumI3OutMin=[]  SumI3OutMax=[]  SumI4OutMin=[]  SumI4OutMax=[]  SumDOutMin=[]  SumDOutMax=[]  DifferentiatorOutMin=[]  DifferentiatorOutMax=[]  FilterDiffOutCoefMin=[]  FilterDiffOutCoefMax=[]  ReciprocalOutMin=[]  ReciprocalOutMax=[]  SumDenOutMin=[]  SumDenOutMax=[]  SumNumOutMin=[]  SumNumOutMax=[]  DivideOutMin=[]  DivideOutMax=[]  UdiffTsProdOutMin=[]  UdiffTsProdOutMax=[]  NTsProdOutMin=[]  NTsProdOutMax=[]  UintegralTsProdOutMin=[]  UintegralTsProdOutMax=[]  UngainTsProdOutMin=[]  UngainTsProdOutMax=[]  ClampingZeroOutDataTypeStr=Inherit: Inherit via back propagation  ClampingZeroOutMin=[]  ClampingZeroOutMax=[]  FilterDenConstantOutDataTypeStr=Inherit: Inherit via back propagation  FilterDenConstantOutMin=[]  FilterDenConstantOutMax=[]  PCopyOutDataTypeStr=Inherit: Inherit via back propagation  PCopyOutMin=[]  PCopyOutMax=[]  NCopyOutDataTypeStr=Inherit: Inherit via back propagation  NCopyOutMin=[]  NCopyOutMax=[]  IntegratorContinuousStateAttributes=''  IntegratorStateMustResolveToSignalObject=off  IntegratorRTWStateStorageClass=Auto  FilterContinuousStateAttributes=''  FilterStateMustResolveToSignalObject=off  FilterRTWStateStorageClass=Auto  ParallelPVariant=InternalParameters  IdealPVariant=Disabled  IVariant=InternalParameters  DVariant=InternalParameters  IntegratorVariant=Continuous  SatVariant=Enabled  AWVariant=BackCalculation  PCopyVariant=Disabled  TRVariant=Disabled  FdbkBlocksVariant=Forward  IdealPFdbkVariant=Disabled  SatFdbkVariant=Disabled  DerivativeFilterVariant=ContFilter  NVariant=InternalParameters  NCopyVariant=Disabled  FilterICVariant=InternalICsFilter  IntegratorICVariant=InternalICs  ExternalResetVariant=Disabled  TRSumVariant=Passthrough  SumFdbkVariant=Disabled  SumVariant=Sum_PID  TsampFilterVariant=InternalTs  TsampNgainVariant=Passthrough  TsampIntegralVariant=Disabled_SignalSpec  ExternalSaturationOutDataTypeStr=Inherit: Same as second input  DerivativeSourceVariant=ErrorSignal  PreIntVariant=InternalPreInt
  Rate Transition : RateTransition
  Rate Transition1 : RateTransition
  f_sw : Constant  Value=50000
  kW_Converter : Gain  Gain=0.001
  n_ratio : Constant  Value=8.2
  I_Low : Outport
  I_High : Outport  Port=2
  tag scope: DAB_Power=global
  wires:
  DAB_Power_Eqn/1(P) -> Calc_I2_avg/1, kW_Converter/1, Calc_I1_avg/1
  Gain/1 -> DAB_Power_Eqn/3(phi)
  Add/1 -> PID Controller/1
  L_lk/1 -> DAB_Power_Eqn/6(L)
  V_High/1 -> Calc_I2_avg/2, DAB_Power_Eqn/2(V2)
  f_sw/1 -> DAB_Power_Eqn/5(f)
  I_High_Ref/1 -> Add/1, Mux/1  "I_DAB_Ref"
  n_ratio/1 -> DAB_Power_Eqn/4(n)
  PID Controller/1 -> Gain/1
  Calc_I2_avg/1 -> I_High/1, Mux/2, Delay/1  "I_DAB_Act"
  Mux/1 -> DAB_Control/1
  kW_Converter/1 -> [DAB_Power]
  Delay/1 -> Rate Transition/1
  V_Low/1 -> Calc_I1_avg/2, DAB_Power_Eqn/1(V1)
  Rate Transition/1 -> Add/2
  Calc_I1_avg/1 -> Delay1/1
  Delay1/1 -> Rate Transition1/1
  Rate Transition1/1 -> I_Low/1

== system INtegrated_Simplified_Batteries_2/Driver ==
  Motor_RPM_Request : Inport
  Motor RPM : Inport  Port=2
  Abs : Abs  SaturateOnIntegerOverflow=off
  Add : Sum  Inputs=+-
  Constant : Constant  Value=30
  Delay : Delay  DelayLength=1
  PID Controller : slpidlib/PID Controller  Controller=PID  Form=Parallel  TimeDomain=Continuous-time  UseExternalTs=off  SampleTime=-1  IntegratorMethod=Forward Euler  FilterMethod=Forward Euler  ControllerParametersSource=internal  P=0.1  I=0.001  UseKiTs=off  D=0.001  UseExternalDerivativeSource=off  N=2.39883291901949  UseFilter=on  TunerSelectOption=Transfer Function Based (PID Tuner App)  InitialConditionSource=internal  InitialConditionForIntegrator=0  InitialConditionForFilter=0  DifferentiatorICPrevScaledInput=0  ExternalReset=either  TrackingMode=off  Kt=0.05  LimitOutput=on  SatLimitsSource=internal  UpperSaturationLimit=400  LowerSaturationLimit=-700  LinearizeAsGain=on  AntiWindupMode=clamping  Kb=1  LimitIntegrator=on  UpperIntegratorSaturationLimit=400  LowerIntegratorSaturationLimit=-700  POutMin=[]  POutMax=[]  IOutMin=[]  IOutMax=[]  DOutMin=[]  DOutMax=[]  NOutMin=[]  NOutMax=[]  SumOutMin=[]  SumOutMax=[]  SaturationOutMin=[]  SaturationOutMax=[]  PParamMin=[]  PParamMax=[]  IParamMin=[]  IParamMax=[]  DParamMin=[]  DParamMax=[]  NParamMin=[]  NParamMax=[]  KbParamMin=[]  KbParamMax=[]  KtParamMin=[]  KtParamMax=[]  KbOutMin=[]  KbOutMax=[]  KtOutMin=[]  KtOutMax=[]  IntegratorOutMin=[]  IntegratorOutMax=[]  FilterOutMin=[]  FilterOutMax=[]  SumI1OutMin=[]  SumI1OutMax=[]  SumI2OutMin=[]  SumI2OutMax=[]  SumI3OutMin=[]  SumI3OutMax=[]  SumI4OutMin=[]  SumI4OutMax=[]  SumDOutMin=[]  SumDOutMax=[]  DifferentiatorOutMin=[]  DifferentiatorOutMax=[]  FilterDiffOutCoefMin=[]  FilterDiffOutCoefMax=[]  ReciprocalOutMin=[]  ReciprocalOutMax=[]  SumDenOutMin=[]  SumDenOutMax=[]  SumNumOutMin=[]  SumNumOutMax=[]  DivideOutMin=[]  DivideOutMax=[]  UdiffTsProdOutMin=[]  UdiffTsProdOutMax=[]  NTsProdOutMin=[]  NTsProdOutMax=[]  UintegralTsProdOutMin=[]  UintegralTsProdOutMax=[]  UngainTsProdOutMin=[]  UngainTsProdOutMax=[]  ClampingZeroOutDataTypeStr=Inherit: Inherit via back propagation  ClampingZeroOutMin=[]  ClampingZeroOutMax=[]  FilterDenConstantOutDataTypeStr=Inherit: Inherit via back propagation  FilterDenConstantOutMin=[]  FilterDenConstantOutMax=[]  PCopyOutDataTypeStr=Inherit: Inherit via back propagation  PCopyOutMin=[]  PCopyOutMax=[]  NCopyOutDataTypeStr=Inherit: Inherit via back propagation  NCopyOutMin=[]  NCopyOutMax=[]  IntegratorContinuousStateAttributes=''  IntegratorStateMustResolveToSignalObject=off  IntegratorRTWStateStorageClass=Auto  FilterContinuousStateAttributes=''  FilterStateMustResolveToSignalObject=off  FilterRTWStateStorageClass=Auto  ParallelPVariant=InternalParameters  IdealPVariant=Disabled  IVariant=InternalParameters  DVariant=InternalParameters  IntegratorVariant=Continuous  SatVariant=Enabled  AWVariant=ContClampingParallel  PCopyVariant=Disabled  TRVariant=Disabled  FdbkBlocksVariant=Forward  IdealPFdbkVariant=Disabled  SatFdbkVariant=Disabled  DerivativeFilterVariant=ContFilter  NVariant=InternalParameters  NCopyVariant=Disabled  FilterICVariant=InternalICsFilter  IntegratorICVariant=InternalICs  ExternalResetVariant=ExternalReset  TRSumVariant=Passthrough  SumFdbkVariant=Disabled  SumVariant=Sum_PID  TsampFilterVariant=InternalTs  TsampNgainVariant=Passthrough  TsampIntegralVariant=Disabled_SignalSpec  ExternalSaturationOutDataTypeStr=Inherit: Same as second input  DerivativeSourceVariant=ErrorSignal  PreIntVariant=InternalPreInt
  Rate Transition : RateTransition
  Relational Operator : RelationalOperator  Operator=<=  OutDataTypeStr=boolean  RndMeth=Simplest  InputSameDT=off
  Driveline_Torque_Request : Outport
  Motor_RPM_Delayed : Outport  Port=2
  wires:
  Rate Transition/1 -> Add/2, Motor_RPM_Delayed/1
  Delay/1 -> Rate Transition/1
  Add/1 -> Abs/1, PID Controller/1
  Motor_RPM_Request/1 -> Add/1
  PID Controller/1 -> Driveline_Torque_Request/1  "Driveline_Torque_Request"
  Motor RPM/1 -> Delay/1
  Relational Operator/1 -> PID Controller/2
  Abs/1 -> Relational Operator/1
  Constant/1 -> Relational Operator/2

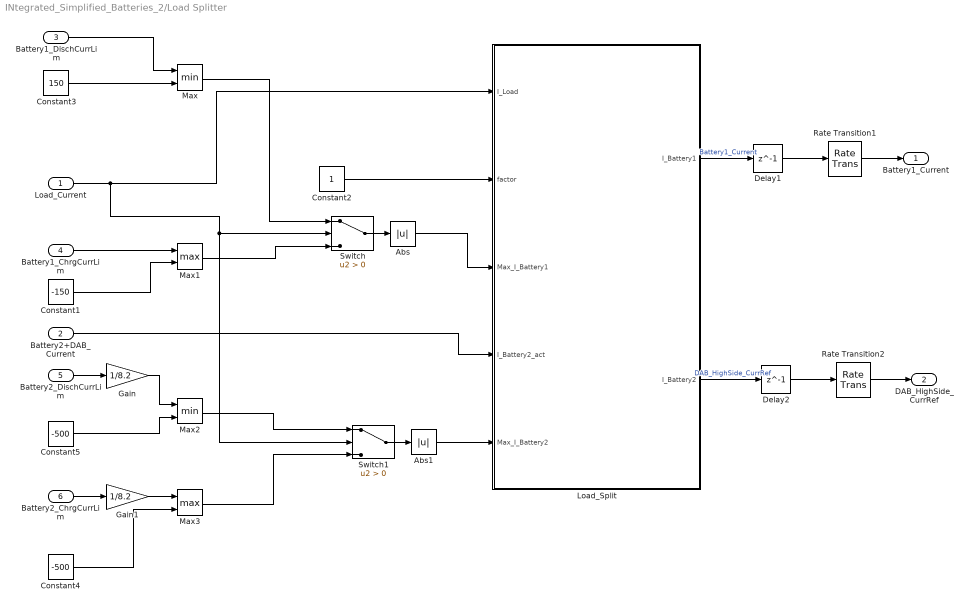
== system INtegrated_Simplified_Batteries_2/Load Splitter ==
  Load_Current : Inport
  Battery2+DAB_Current : Inport  Port=2
  Battery1_DischCurrLim : Inport  Port=3
  Battery1_ChrgCurrLim : Inport  Port=4
  Battery2_DischCurrLim : Inport  Port=5
  Battery2_ChrgCurrLim : Inport  Port=6
  Abs : Abs  SaturateOnIntegerOverflow=off
  Abs1 : Abs  SaturateOnIntegerOverflow=off
  Constant1 : Constant  Value=-150
  Constant2 : Constant
  Constant3 : Constant  Value=150
  Constant4 : Constant  Value=-500
  Constant5 : Constant  Value=-500
  Delay1 : Delay  DelayLength=1
  Delay2 : Delay  DelayLength=1
  Gain : Gain  Gain=1/8.2
  Gain1 : Gain  Gain=1/8.2
  Load_Split : MATLAB Function  TreatAsAtomicUnit=on
  Max : MinMax  Inputs=2
  Max1 : MinMax  Function=max  Inputs=2
  Max2 : MinMax  Inputs=2
  Max3 : MinMax  Function=max  Inputs=2
  Rate Transition1 : RateTransition
  Rate Transition2 : RateTransition
  Switch : Switch  Criteria=u2 > Threshold  SaturateOnIntegerOverflow=off  InputSameDT=off
  Switch1 : Switch  Criteria=u2 > Threshold  SaturateOnIntegerOverflow=off  InputSameDT=off
  Battery1_Current : Outport
  DAB_HighSide_CurrRef : Outport  Port=2
  wires:
  Max/1 -> Switch/1
  Battery1_ChrgCurrLim/1 -> Max1/1
  Constant3/1 -> Max/2
  Delay1/1 -> Rate Transition1/1
  Max1/1 -> Switch/3
  Rate Transition1/1 -> Battery1_Current/1
  Delay2/1 -> Rate Transition2/1
  Rate Transition2/1 -> DAB_HighSide_CurrRef/1
  Load_Split/2(I_Battery2) -> Delay2/1  "DAB_HighSide_CurrRef"
  Switch/1 -> Abs/1
  Load_Split/1(I_Battery1) -> Delay1/1  "Battery1_Current"
  Constant2/1 -> Load_Split/2(factor)
  Abs/1 -> Load_Split/3(Max_I_Battery1)
  Constant1/1 -> Max1/2
  Battery1_DischCurrLim/1 -> Max/1
  Battery2+DAB_Current/1 -> Load_Split/4(I_Battery2_act)
  Battery2_DischCurrLim/1 -> Gain/1
  Battery2_ChrgCurrLim/1 -> Gain1/1
  Gain/1 -> Max2/1
  Constant4/1 -> Max3/2
  Load_Current/1 -> Load_Split/1(I_Load), Switch1/2, Switch/2
  Switch1/1 -> Abs1/1
  Max3/1 -> Switch1/3
  Constant5/1 -> Max2/2
  Gain1/1 -> Max3/1
  Max2/1 -> Switch1/1
  Abs1/1 -> Load_Split/5(Max_I_Battery2)

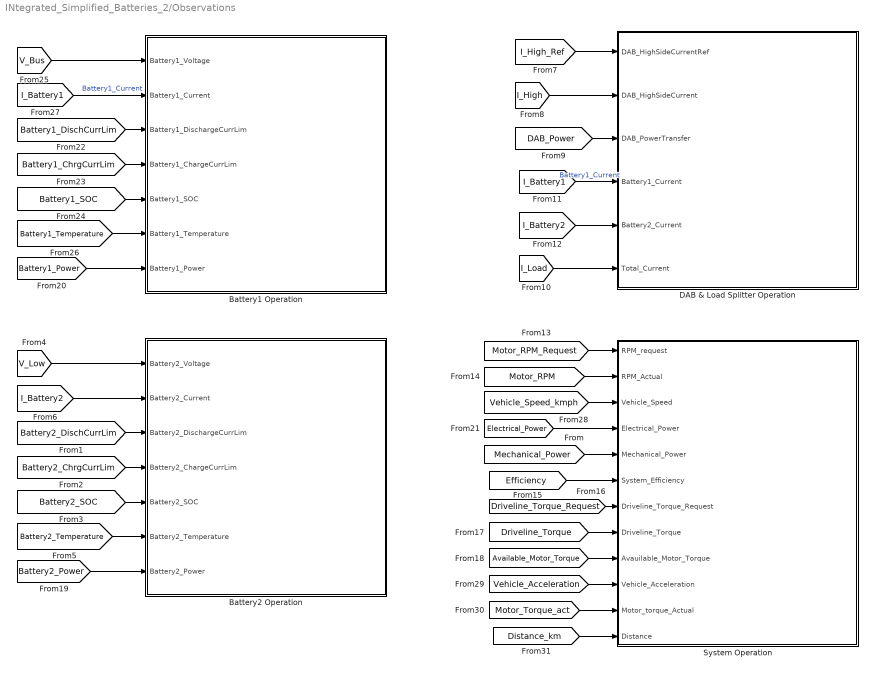
== system INtegrated_Simplified_Batteries_2/Observations ==
  Battery1 Operation : Subsystem
  Battery2 Operation : Subsystem
  DAB & Load Splitter Operation : Subsystem
  System Operation : Subsystem
  wires:
  [V_Bus] -> Battery1 Operation/1(Battery1_Voltage)
  [I_Battery1] -> Battery1 Operation/2(Battery1_Current)  "Battery1_Current"
  [Battery1_DischCurrLim] -> Battery1 Operation/3(Battery1_DischargeCurrLim)
  [Battery1_ChrgCurrLim] -> Battery1 Operation/4(Battery1_ChargeCurrLim)
  [Battery1_SOC] -> Battery1 Operation/5(Battery1_SOC)
  [Battery1_Temperature] -> Battery1 Operation/6(Battery1_Temperature)
  [Battery2_DischCurrLim] -> Battery2 Operation/3(Battery2_DischargeCurrLim)
  [Battery2_ChrgCurrLim] -> Battery2 Operation/4(Battery2_ChargeCurrLim)
  [Battery2_SOC] -> Battery2 Operation/5(Battery2_SOC)
  [Battery2_Temperature] -> Battery2 Operation/6(Battery2_Temperature)
  [I_Battery2] -> Battery2 Operation/2(Battery2_Current)
  [V_Low] -> Battery2 Operation/1(Battery2_Voltage)
  [I_High_Ref] -> DAB & Load Splitter Operation/1(DAB_HighSideCurrentRef)
  [DAB_Power] -> DAB & Load Splitter Operation/3(DAB_PowerTransfer)
  [I_High] -> DAB & Load Splitter Operation/2(DAB_HighSideCurrent)
  [I_Load] -> DAB & Load Splitter Operation/6(Total_Current)
  [I_Battery1] -> DAB & Load Splitter Operation/4(Battery1_Current)  "Battery1_Current"
  [I_Battery2] -> DAB & Load Splitter Operation/5(Battery2_Current)
  [Motor_RPM_Request] -> System Operation/1(RPM_request)
  [Motor_RPM] -> System Operation/2(RPM_Actual)
  [Efficiency] -> System Operation/6(System_Efficiency)
  [Driveline_Torque_Request] -> System Operation/7(Driveline_Torque_Request)
  [Driveline_Torque] -> System Operation/8(Driveline_Torque)
  [Available_Motor_Torque] -> System Operation/9(Avauilable_Motor_Torque)
  [Battery2_Power] -> Battery2 Operation/7(Battery2_Power)
  [Battery1_Power] -> Battery1 Operation/7(Battery1_Power)
  [Electrical_Power] -> System Operation/4(Electrical_Power)
  [Mechanical_Power] -> System Operation/5(Mechanical_Power)
  [Vehicle_Speed_kmph] -> System Operation/3(Vehicle_Speed)
  [Vehicle_Acceleration] -> System Operation/10(Vehicle_Acceleration)
  [Motor_Torque_act] -> System Operation/11(Motor_torque_Actual)
  [Distance_km] -> System Operation/12(Distance)
